simulink model "PSC"  (R2016b)
settings: Solver=VariableStepAuto  StartTime=0.0  StopTime=5  RelTol=1e-3
values from neighbouring files (symbols this model uses):
  A = 1.3    [PV_module_Code.m]
  Isc = 8.61    [PV_module_Code.m]
  Ki = 0.002    [PV_module_Code.m]
  Kv = -0.32    [PV_module_Code.m]
  Ns = 60    [PV_module_Code.m]
  Rp = 415    [PV_module_Code.m]
  Rs = 0.22    [PV_module_Code.m]
  Voc = 37.41    [PV_module_Code.m]
undefined symbols (not defined in the file or in its folder): sigbuilder_block
libraries: powerlib x26, powerlib_meascontrol x1, fuzblock x1
settings Model: Creator=adria  LastModifiedBy=adria
settings DebuggingCC: UnconnectedInputMsg=none  UnconnectedOutputMsg=none  UnconnectedLineMsg=none

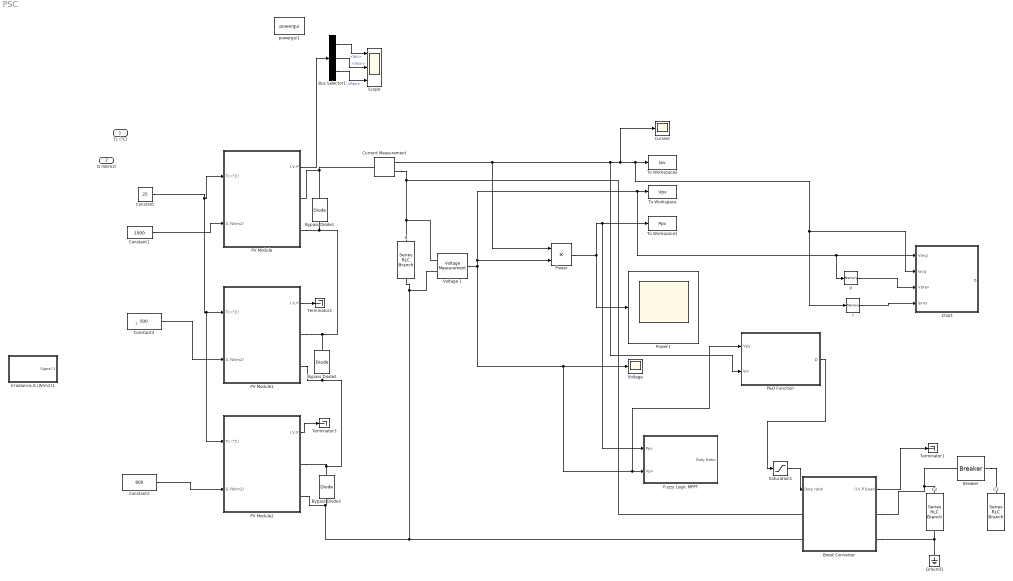
== system PSC ==
  note: 1
  Tc (°C) : Inport
  G (W/m2) : Inport  Port=2
  Boost Converter : Subsystem
  Breaker : powerlib/Elements/Breaker  InitialState=0  SwitchingTimes=[7]  External=off  BreakerResistance=0.00001  SnubberResistance=1e6  SnubberCapacitance=inf  Measurements=None  MoreParameters=on  NoBreakLoop=off
  Bus Selector1 : BusSelector  OutputSignals=Ipv,Vpv,Ppv
  Bypass Diode1 : powerlib/Power Electronics/Diode  Ron=0.00001  Lon=0  Vf=0.8  IC=0  UseSnubber=off  Rs=500  Cs=250e-9  Measurements=off
  Bypass Diode2 : powerlib/Power Electronics/Diode  Ron=0.00001  Lon=0  Vf=0.8  IC=0  UseSnubber=off  Rs=500  Cs=250e-9  Measurements=off
  Bypass Diode3 : powerlib/Power Electronics/Diode  Ron=0.00001  Lon=0  Vf=0.8  IC=0  UseSnubber=off  Rs=500  Cs=250e-9  Measurements=off
  C : powerlib/Elements/Series RLC Branch  LConnTagsString=__new0  RConnTagsString=__new0  BranchType=C  Resistance=3.7  Inductance=1e-3  SetiL0=off  InitialCurrent=0  Capacitance=50e-4  Setx0=off  InitialVoltage=0  Measurements=Branch voltage
  C2 : powerlib/Elements/Series RLC Branch  LConnTagsString=__new0  RConnTagsString=__new0  BranchType=R  Resistance=10  Inductance=1e-3  SetiL0=off  InitialCurrent=0  Capacitance=19e-4  Setx0=off  InitialVoltage=0  Measurements=Branch voltage
  C3 : powerlib/Elements/Series RLC Branch  LConnTagsString=__new0  RConnTagsString=__new0  BranchType=R  Resistance=100  Inductance=1e-3  SetiL0=off  InitialCurrent=0  Capacitance=19e-4  Setx0=off  InitialVoltage=0  Measurements=Branch voltage
  Chart : Stateflow chart  TreatAsAtomicUnit=on
  Constant : Constant  Value=25
  Constant1 : Constant  Value=1000
  Constant2 : Constant  Value=800
  Constant3 : Constant  Value=500
  Current : Scope
  Current Measurement : powerlib/Measurements/Current Measurement  PhasorSimulation=off  OutputType=Complex  PSBequivalent=0
  Fuzzy Logic MPPT : Subsystem
  Ground1 : powerlib/Elements/Ground  LConnTagsString=a
  I : Memory
  Irradiance,G (W/m2)1 : Subsystem  Tag=STV Subsys  LoadFcn=sigbuilder_block('load');  StartFcn=sigbuilder_block('start');  StopFcn=sigbuilder_block('stop');  ClipboardFcn=sigbuilder_block('clipboard');  mask(Sigbuilder block){tuvar=[0:10]}
      mask help: Simulink:masks:SigbuilderBlock_MD
      mask init:
      | if ~strcmp(get_param(bdroot(gcbh),'SimulationStatus'),'stopped') tuvar = sigbuilder_block('maskInit'); end
      settings: CopyFcn=sigbuilder_block('copy');  DeleteFcn=sigbuilder_block('delete');  ModelCloseFcn=sigbuilder_block('modelClose');  PreSaveFcn=sigbuilder_block('preSave');  PauseFcn=sigbuilder_block('pause');  ContinueFcn=sigbuilder_block('continue');  NameChangeFcn=sigbuilder_block('namechange');  OpenFcn=sigbuilder_block('open',[484.8 30.6 470.4 453 ]);  CloseFcn=sigbuilder_block('close');
      mask Display: plot(0, 0, 100, 100,[2, 2, 32, 32, 2], [68, 8, 8, 68, 68],[32, 2], [38, 38], [32, 19, 2],[53, 60, 44], [32, 17, 17, 2],[16, 16, 31, 31]);txt = getActiveGroup(gcbh);text(2, 100, txt,'verticalAlignment', 'top');
  P&O Function : MATLAB Function  TreatAsAtomicUnit=on
  PV Module : Subsystem
  PV Module1 : Subsystem
  PV Module2 : Subsystem
  Power : Product
  Power1 : Scope
  Saturation1 : Saturate  UpperLimit=1  LowerLimit=0.001  ZeroCross=off
  Scope : Scope  NumInputPorts=3
  Terminator1 : Terminator
  Terminator2 : Terminator
  Terminator3 : Terminator
  To Workspace : ToWorkspace  VariableName=Vpv  SampleTime=-1
  To Workspace1 : ToWorkspace  VariableName=Ppv  SampleTime=-1
  To Workspace2 : ToWorkspace  VariableName=Ipv  SampleTime=-1
  V : Memory
  Voltage : Scope
  Voltage 1 : powerlib/Measurements/Voltage Measurement  PhasorSimulation=off  OutputType=Complex  PSBequivalent=0
  powergui1 : powerlib/powergui  Priority=1  SimulationMode=Discrete  SolverType=Tustin/Backward Euler (TBE)  SampleTime=0.00001  frequency=60  SPID=off  DisableSnubberDevices=off  DisableRonSwitches=off  DisableVfSwitches=off  SwTol=0  DisplayEquations=off  Interpol=off  ExternalGateDelay=off  methode=off  Ts=10  FunctionMessages=off  echomessages=off  HookPort=off  EnableUseOfTLC=off  x0status=blocks  frequencyindice=0  Pbase=100e6  ErrMax=1e-4  Iterations=50  UnitsV=kV  UnitsW=MW  buscounter=0  RestoreLinks=warning  ResistiveCurrentMeasurement=off  Frange=[0:2:500]  Ylog=off  Xlog=on  ShowGrid=off  save=off  variable=ZData  structure=0  ZoomFFT=off  StartTime=0.0  cycles=1  DisplayStyle=1  fundamental=60  FreqAxis=off  MaxFrequency=1000  frequencyindicesteady=1  RmsSteady=1  display=off
  wires:
  PV Module/1(I,V,P) -> Bus Selector1/1
  Constant/1 -> PV Module2/1(Tc (°C)), PV Module1/1(Tc (°C)), PV Module/1(Tc (°C))
  Constant1/1 -> PV Module/2(G (W/m2))
  Bus Selector1/2 -> Scope/2  "<Vpv>"
  Bus Selector1/3 -> Scope/3  "<Ppv>"
  Bus Selector1/1 -> Scope/1  "<Ipv>"
  PV Module1/1(I,V,P) -> Terminator2/1
  Current Measurement/1 -> Power/1, P&O Function/2(Ipv), Current/1, Chart/2(Iavg), I/1, To Workspace2/1
  Boost Converter/1((I,V,P)Load) -> Terminator1/1
  Power/1 -> Fuzzy Logic MPPT/1(Ppv), To Workspace1/1, Power1/1
  V/1 -> Chart/3(Vprev)
  I/1 -> Chart/4(Iprev)
  Voltage 1/1 -> Power/2, Chart/1(Vavg), V/1, To Workspace/1, P&O Function/1(Vpv), Fuzzy Logic MPPT/2(Vpv), Voltage/1
  Constant3/1 -> PV Module1/2(G (W/m2))
  PV Module2/1(I,V,P) -> Terminator3/1
  Constant2/1 -> PV Module2/2(G (W/m2))
  Saturation1/1 -> Boost Converter/1("Duty ratio ")
  P&O Function/1(D) -> Saturation1/1
  connections:
  PV Module/RConn2 -- Bypass Diode1/LConn1 -- Bypass Diode2/RConn1 -- PV Module1/RConn1
  PV Module/RConn1 -- Bypass Diode1/RConn1 -- Current Measurement/LConn1
  Voltage 1/LConn1 -- Boost Converter/LConn1 -- Current Measurement/RConn1 -- C/LConn1
  Boost Converter/RConn2 -- C2/RConn1 -- Ground1/LConn1
  Boost Converter/RConn1 -- Breaker/LConn1 -- C2/LConn1
  Breaker/RConn1 -- C3/LConn1
  PV Module2/RConn2 -- Boost Converter/LConn2 -- Voltage 1/LConn2 -- C/RConn1 -- Bypass Diode3/LConn1
  PV Module2/RConn1 -- Bypass Diode2/LConn1 -- PV Module1/RConn2 -- Bypass Diode3/RConn1

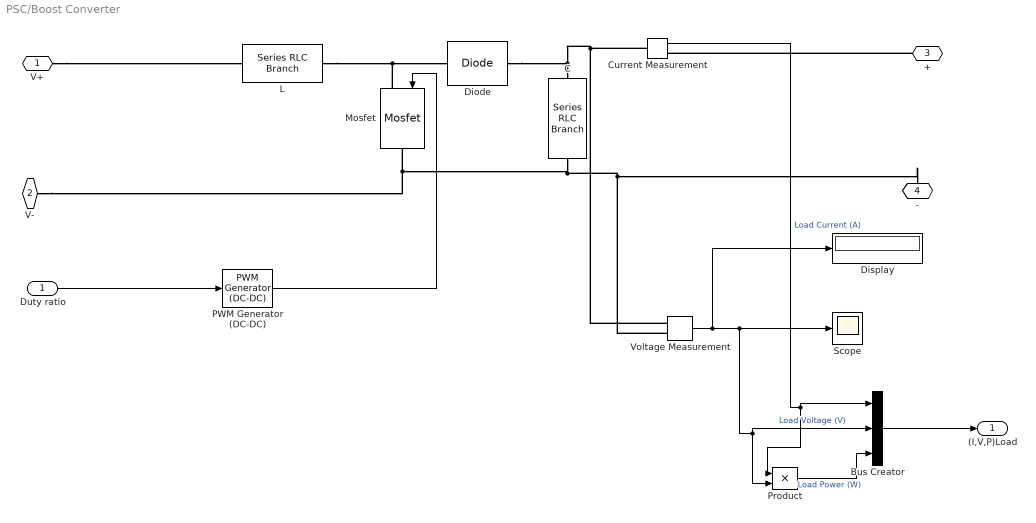
== system PSC/Boost Converter ==
  "Duty ratio " : Inport
  Bus Creator : BusCreator  Inputs='Load Current (A)','Load Voltage (V)','Load Power (W)'
  C : powerlib/Elements/Series RLC Branch  LConnTagsString=__new0  RConnTagsString=__new0  BranchType=C  Resistance=1  Inductance=1e-3  SetiL0=off  InitialCurrent=0  Capacitance=80e-7  Setx0=off  InitialVoltage=0  Measurements=None
  Current Measurement : powerlib/Measurements/Current Measurement  PhasorSimulation=off  OutputType=Complex  PSBequivalent=0
  Diode : powerlib/Power Electronics/Diode  Ron=0.0001  Lon=0  Vf=0.8  IC=0  UseSnubber=off  Rs=500  Cs=250e-9  Measurements=off
  Display : Display
  L : powerlib/Elements/Series RLC Branch  LConnTagsString=__new0  RConnTagsString=__new0  BranchType=L  Resistance=1  Inductance=1e-3  SetiL0=off  InitialCurrent=0  Capacitance=1e-6  Setx0=off  InitialVoltage=0  Measurements=None
  Mosfet : powerlib/Power Electronics/Mosfet  Ron=0.0001  Lon=0  Rd=0.0001  Vfd=0  IC=0  Rs=1e5  Cs=inf  Measurements=off
  PWM Generator (DC-DC) : powerlib_meascontrol/Pulse & Signal Generators/PWM Generator (DC-DC)  Fsw=1000  Ts=0
  Product : Product
  Scope : Scope
  Voltage Measurement : powerlib/Measurements/Voltage Measurement  PhasorSimulation=off  OutputType=Complex  PSBequivalent=0
  V+ : PMIOPort  Port=1  Side=Left
  V- : PMIOPort  Port=2  Side=Left
  + : PMIOPort  Port=3  Side=Right
  - : PMIOPort  Port=4  Side=Right
  (I,V,P)Load : Outport
  wires:
  PWM Generator (DC-DC)/1 -> Mosfet/1
  Voltage Measurement/1 -> Display/1, Product/2, Bus Creator/2, Scope/1  "Load Voltage (V)"
  "Duty ratio "/1 -> PWM Generator (DC-DC)/1
  Current Measurement/1 -> Product/1, Bus Creator/1  "Load Current (A)"
  Product/1 -> Bus Creator/3  "Load Power (W)"
  Bus Creator/1 -> (I,V,P)Load/1
  connections:
  V+/RConn1 -- L/LConn1
  L/RConn1 -- Mosfet/LConn1 -- Diode/LConn1
  +/RConn1 -- Current Measurement/RConn1
  -/RConn1 -- Voltage Measurement/LConn2 -- V-/RConn1 -- Mosfet/RConn1 -- C/RConn1
  Diode/RConn1 -- Current Measurement/LConn1 -- Voltage Measurement/LConn1 -- C/LConn1

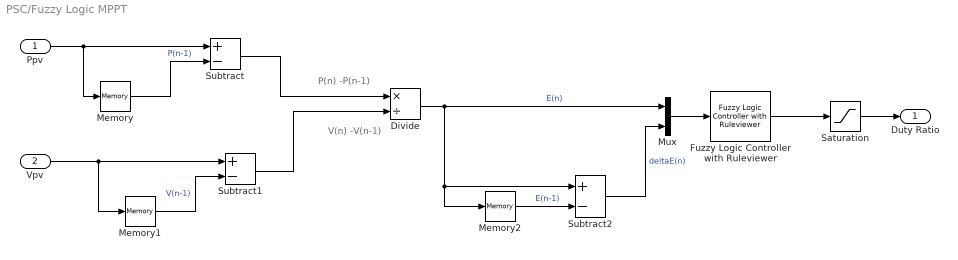
== system PSC/Fuzzy Logic MPPT ==
  note: P(n) -P(n-1)
  note: V(n) -V(n-1)
  Ppv : Inport
  Vpv : Inport  Port=2
  Divide : Product  Inputs=*/
  Fuzzy Logic Controller with Ruleviewer : fuzblock/Fuzzy Logic  Controller  with Ruleviewer  fismatrix=MPPT7  Ts=1
  Memory : Memory
  Memory1 : Memory
  Memory2 : Memory
  Mux : Mux  Inputs=2
  Saturation : Saturate  UpperLimit=1  LowerLimit=0  LinearizeAsGain=off  ZeroCross=off
  Subtract : Sum  Inputs=+-
  Subtract1 : Sum  Inputs=+-
  Subtract2 : Sum  Inputs=+-
  Duty Ratio : Outport
  wires:
  Ppv/1 -> Subtract/1, Memory/1
  Mux/1 -> Fuzzy Logic Controller with Ruleviewer/1
  Divide/1 -> Subtract2/1, Memory2/1, Mux/1  "E(n)"
  Memory2/1 -> Subtract2/2  "E(n-1)"
  Subtract2/1 -> Mux/2  "deltaE(n)"
  Memory/1 -> Subtract/2  "P(n-1)"
  Vpv/1 -> Memory1/1, Subtract1/1
  Memory1/1 -> Subtract1/2  "V(n-1)"
  Saturation/1 -> Duty Ratio/1
  Subtract1/1 -> Divide/2
  Subtract/1 -> Divide/1
  Fuzzy Logic Controller with Ruleviewer/1 -> Saturation/1

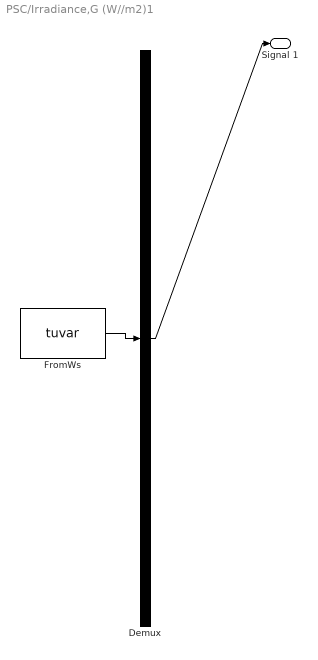
== system PSC/Irradiance,G (W//m2)1 ==
  Demux : Demux  Tag=STV Demux  Outputs=1
  FromWs : FromWorkspace  Tag=STV FromWs  VariableName=tuvar  SampleTime=0
      SigBuilderData=|
      | common.afterFinalStr = 'Extrapolate'
      | common.sampleTime = 0
      | dataSet.timeRange = [0 10]
      | dataSet.name = 'Irradiance Variation Pattern'
      | sbobj.Groups.Name = 'Irradiance Variation Pattern'
      | sbobj.Groups.Signals.Name = 'Signal 1'
      | sbobj.Groups.Signals.XData = [0 0.2 0.2 0.3 0.3 0.8 0.8 0.9 2.4 2.4 3.6 3.6 10]
      | sbobj.Groups.Signals.YData = [1000 1000 300 300 1000 1000 995 995 995 575 1 0 0]
  Signal 1 : Outport  Tag=STV Outport
  wires:
  FromWs/1 -> Demux/1
  Demux/1 -> Signal 1/1

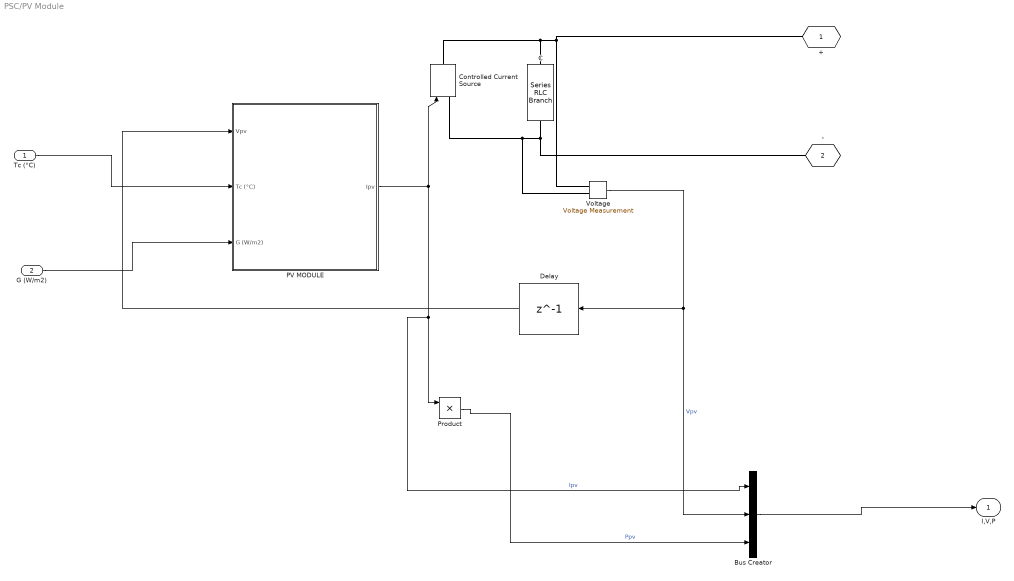
== system PSC/PV Module ==
  Tc (°C) : Inport
  G (W/m2) : Inport  Port=2
  Bus Creator : BusCreator  Inputs='Ipv','Vpv','Ppv'
  C : powerlib/Elements/Series RLC Branch  LConnTagsString=__new0  RConnTagsString=__new0  BranchType=C  Resistance=10  Inductance=1e-3  SetiL0=off  InitialCurrent=0  Capacitance=25e-6  Setx0=off  InitialVoltage=0  Measurements=Branch voltage
  Controlled Current Source : powerlib/Electrical Sources/Controlled Current Source  Initialize=on  Source_Type=AC  Amplitude=0  Phase=0  Frequency=0  Measurements=None
  Delay : Delay  DelayLength=1  InitialCondition=0
  PV MODULE : Subsystem
  Product : Product
  "Voltage " : powerlib/Measurements/Voltage Measurement  PhasorSimulation=off  OutputType=Complex  PSBequivalent=0
  + : PMIOPort  Port=1  Side=Right
  - : PMIOPort  Port=2  Side=Right
  I,V,P : Outport
  wires:
  Product/1 -> Bus Creator/3  "Ppv"
  Tc (°C)/1 -> PV MODULE/2("Tc (°C) ")
  G (W/m2)/1 -> PV MODULE/3(G (W/m2))
  "Voltage "/1 -> Bus Creator/2, Delay/1  "Vpv"
  PV MODULE/1(Ipv) -> Controlled Current Source/1, Bus Creator/1, Product/1  "Ipv"
  Bus Creator/1 -> I,V,P/1
  Delay/1 -> PV MODULE/1(Vpv)
  connections:
  Controlled Current Source/LConn1 -- -/RConn1 -- C/RConn1 -- "Voltage "/LConn2
  Controlled Current Source/RConn1 -- C/LConn1 -- +/RConn1 -- "Voltage "/LConn1

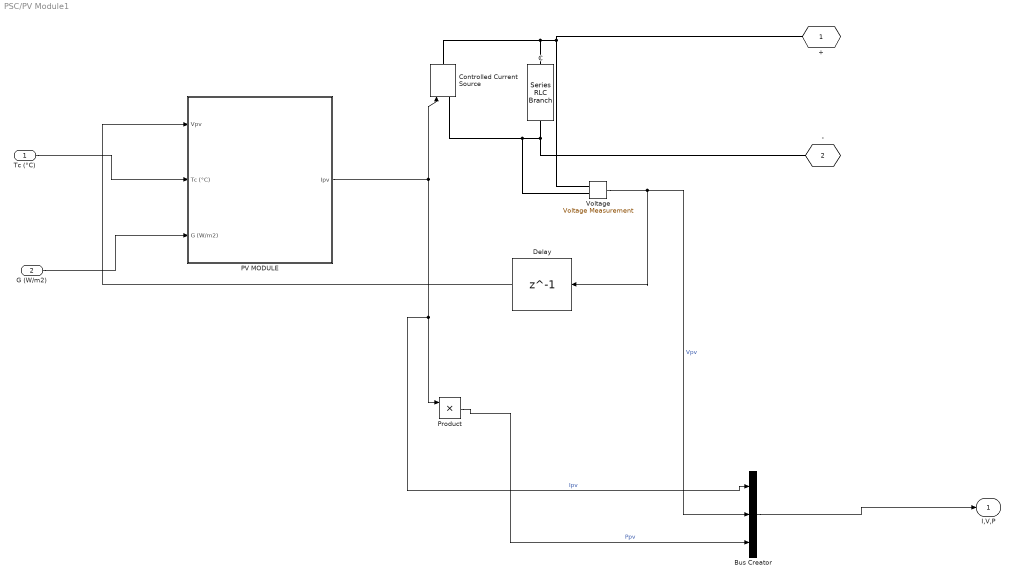
== system PSC/PV Module1 ==
  Tc (°C) : Inport
  G (W/m2) : Inport  Port=2
  Bus Creator : BusCreator  Inputs='Ipv','Vpv','Ppv'
  C : powerlib/Elements/Series RLC Branch  LConnTagsString=__new0  RConnTagsString=__new0  BranchType=C  Resistance=10  Inductance=1e-3  SetiL0=off  InitialCurrent=0  Capacitance=25e-6  Setx0=off  InitialVoltage=0  Measurements=Branch voltage
  Controlled Current Source : powerlib/Electrical Sources/Controlled Current Source  Initialize=on  Source_Type=AC  Amplitude=0  Phase=0  Frequency=0  Measurements=None
  Delay : Delay  DelayLength=1  InitialCondition=0
  PV MODULE : Subsystem
  Product : Product
  "Voltage " : powerlib/Measurements/Voltage Measurement  PhasorSimulation=off  OutputType=Complex  PSBequivalent=0
  + : PMIOPort  Port=1  Side=Right
  - : PMIOPort  Port=2  Side=Right
  I,V,P : Outport
  wires:
  Product/1 -> Bus Creator/3  "Ppv"
  Tc (°C)/1 -> PV MODULE/2("Tc (°C) ")
  G (W/m2)/1 -> PV MODULE/3(G (W/m2))
  "Voltage "/1 -> Delay/1, Bus Creator/2  "Vpv"
  PV MODULE/1(Ipv) -> Bus Creator/1, Product/1, Controlled Current Source/1  "Ipv"
  Bus Creator/1 -> I,V,P/1
  Delay/1 -> PV MODULE/1(Vpv)
  connections:
  Controlled Current Source/LConn1 -- -/RConn1 -- C/RConn1 -- "Voltage "/LConn2
  Controlled Current Source/RConn1 -- C/LConn1 -- +/RConn1 -- "Voltage "/LConn1

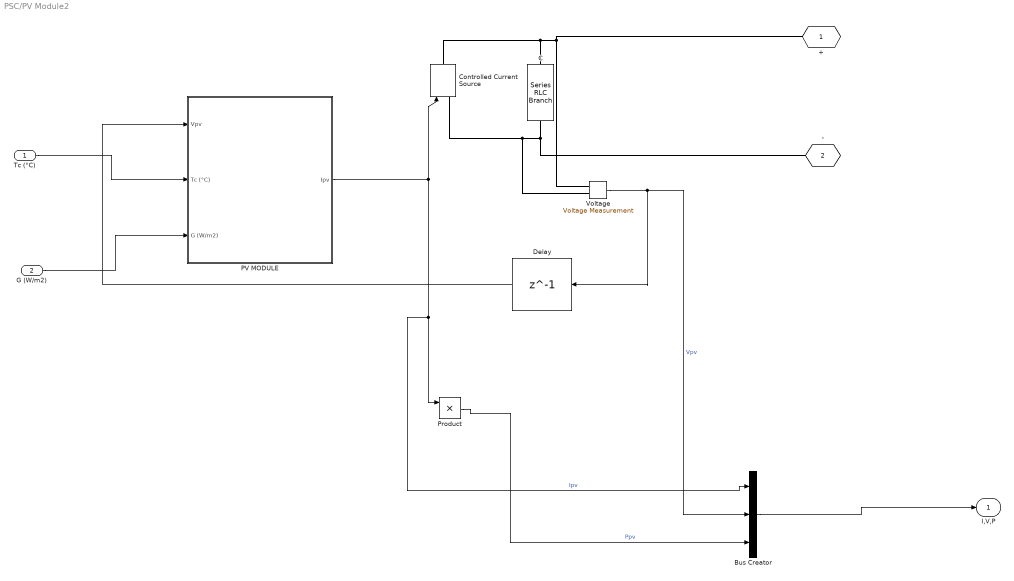
== system PSC/PV Module2 ==
  Tc (°C) : Inport
  G (W/m2) : Inport  Port=2
  Bus Creator : BusCreator  Inputs='Ipv','Vpv','Ppv'
  C : powerlib/Elements/Series RLC Branch  LConnTagsString=__new0  RConnTagsString=__new0  BranchType=C  Resistance=10  Inductance=1e-3  SetiL0=off  InitialCurrent=0  Capacitance=25e-6  Setx0=off  InitialVoltage=0  Measurements=Branch voltage
  Controlled Current Source : powerlib/Electrical Sources/Controlled Current Source  Initialize=on  Source_Type=AC  Amplitude=0  Phase=0  Frequency=0  Measurements=None
  Delay : Delay  DelayLength=1  InitialCondition=0
  PV MODULE : Subsystem
  Product : Product
  "Voltage " : powerlib/Measurements/Voltage Measurement  PhasorSimulation=off  OutputType=Complex  PSBequivalent=0
  + : PMIOPort  Port=1  Side=Right
  - : PMIOPort  Port=2  Side=Right
  I,V,P : Outport
  wires:
  Product/1 -> Bus Creator/3  "Ppv"
  Tc (°C)/1 -> PV MODULE/2("Tc (°C) ")
  G (W/m2)/1 -> PV MODULE/3(G (W/m2))
  "Voltage "/1 -> Delay/1, Bus Creator/2  "Vpv"
  PV MODULE/1(Ipv) -> Bus Creator/1, Product/1, Controlled Current Source/1  "Ipv"
  Bus Creator/1 -> I,V,P/1
  Delay/1 -> PV MODULE/1(Vpv)
  connections:
  Controlled Current Source/LConn1 -- -/RConn1 -- C/RConn1 -- "Voltage "/LConn2
  Controlled Current Source/RConn1 -- C/LConn1 -- +/RConn1 -- "Voltage "/LConn1

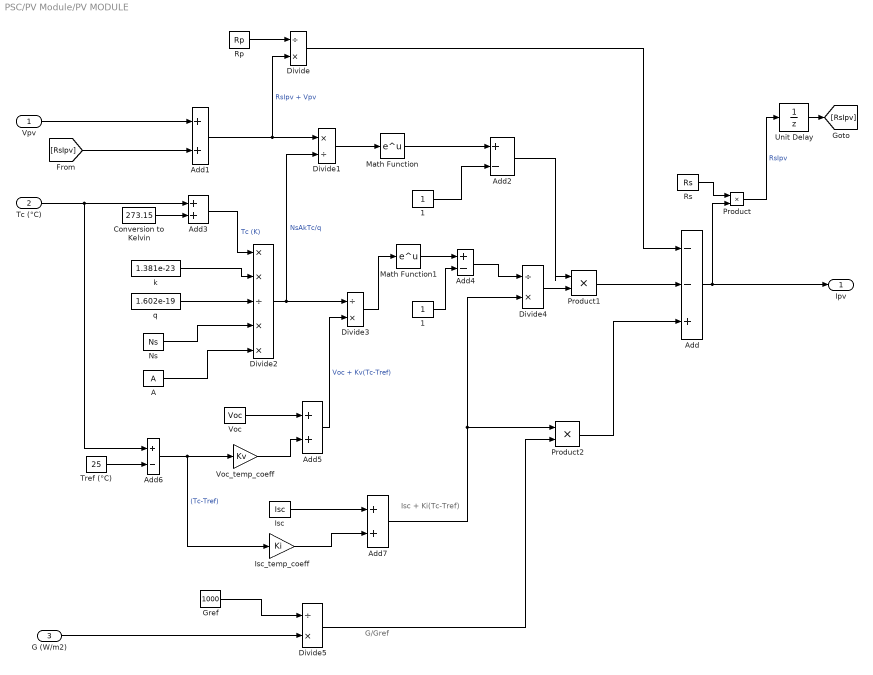
== system PSC/PV Module/PV MODULE ==
  note: G/Gref
  note: Isc + Ki(Tc-Tref)
  Vpv : Inport
  "Tc (°C) " : Inport  Port=2
  G (W/m2) : Inport  Port=3
  " 1" : Constant
  " Gref " : Constant  Value=1000
  " Tref (°C)" : Constant  Value=25
  " Voc" : Constant  Value=Voc
  1 : Constant
  A : Constant  Value=A
  Add : Sum  Inputs=--+
  Add{1,3,5,7} (4 alike) : Sum
  Add2 : Sum  Inputs=+-
  Add4 : Sum  Inputs=+-
  Add6 : Sum  Inputs=+-
  Conversion to Kelvin : Constant  Value=273.15
  Divide{,3..5} (4 alike) : Product  Inputs=/*
  Divide1 : Product  Inputs=*/
  Divide2 : Product  Inputs=**/**
  Isc : Constant  Value=Isc
  "Isc_temp_coeff " : Gain  Gain=Ki
  Math Function : Math  SaturateOnIntegerOverflow=on
  Math Function1 : Math  SaturateOnIntegerOverflow=on
  Ns : Constant  Value=Ns
  Product : Product
  Product1 : Product
  Product2 : Product
  Rp : Constant  Value=Rp
  Rs : Constant  Value=Rs
  Unit Delay : UnitDelay  SampleTime=-1
  Voc_temp_coeff : Gain  Gain=Kv
  k : Constant  Value=1.381e-23
  "q " : Constant  Value=1.602e-19
  Ipv : Outport
  wires:
  A/1 -> Divide2/5
  Vpv/1 -> Add1/1
  Rp/1 -> Divide/1
  Add/1 -> Ipv/1, Product/2
  Product/1 -> Unit Delay/1  "RsIpv"
  Divide/1 -> Add/1
  Add1/1 -> Divide1/1, Divide/2  "RsIpv + Vpv"
  Rs/1 -> Product/1
  Product2/1 -> Add/3
  Divide2/1 -> Divide3/1, Divide1/2  "NsAkTc/q"
  k/1 -> Divide2/2
  Math Function1/1 -> Add4/1
  " Voc"/1 -> Add5/1
  Divide4/1 -> Product1/2
  Add2/1 -> Product1/1
  Math Function/1 -> Add2/1
  Divide3/1 -> Math Function1/1
  "q "/1 -> Divide2/3
  Add6/1 -> "Isc_temp_coeff "/1, Voc_temp_coeff/1  "(Tc-Tref)"
  " 1"/1 -> Add4/2
  Isc/1 -> Add7/1
  Add7/1 -> Product2/1, Divide4/2
  "Tc (°C) "/1 -> Add6/1, Add3/1
  Add4/1 -> Divide4/1
  Product1/1 -> Add/2
  Divide5/1 -> Product2/2
  Conversion to Kelvin/1 -> Add3/2
  Add5/1 -> Divide3/2  "Voc + Kv(Tc-Tref)"
  "Isc_temp_coeff "/1 -> Add7/2
  Divide1/1 -> Math Function/1
  " Gref "/1 -> Divide5/1
  " Tref (°C)"/1 -> Add6/2
  G (W/m2)/1 -> Divide5/2
  Voc_temp_coeff/1 -> Add5/2
  Add3/1 -> Divide2/1  "Tc (K)"
  Ns/1 -> Divide2/4
  1/1 -> Add2/2
  [RsIpv] -> Add1/2
  Unit Delay/1 -> [RsIpv]

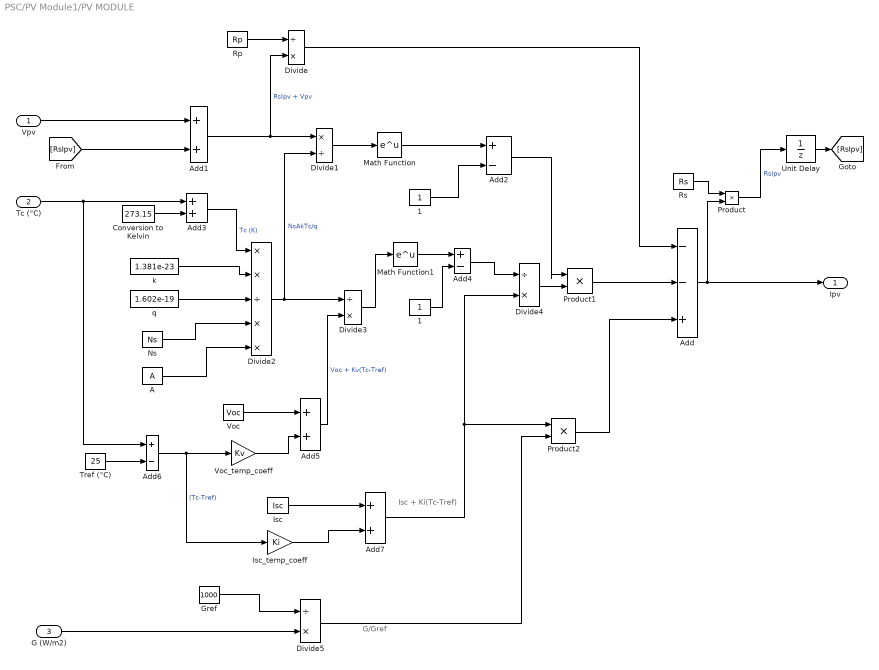
== system PSC/PV Module1/PV MODULE ==
  note: G/Gref
  note: Isc + Ki(Tc-Tref)
  Vpv : Inport
  "Tc (°C) " : Inport  Port=2
  G (W/m2) : Inport  Port=3
  " 1" : Constant
  " Gref " : Constant  Value=1000
  " Tref (°C)" : Constant  Value=25
  " Voc" : Constant  Value=Voc
  1 : Constant
  A : Constant  Value=A
  Add : Sum  Inputs=--+
  Add{1,3,5,7} (4 alike) : Sum
  Add2 : Sum  Inputs=+-
  Add4 : Sum  Inputs=+-
  Add6 : Sum  Inputs=+-
  Conversion to Kelvin : Constant  Value=273.15
  Divide{,3..5} (4 alike) : Product  Inputs=/*
  Divide1 : Product  Inputs=*/
  Divide2 : Product  Inputs=**/**
  Isc : Constant  Value=Isc
  "Isc_temp_coeff " : Gain  Gain=Ki
  Math Function : Math  SaturateOnIntegerOverflow=on
  Math Function1 : Math  SaturateOnIntegerOverflow=on
  Ns : Constant  Value=Ns
  Product : Product
  Product1 : Product
  Product2 : Product
  Rp : Constant  Value=Rp
  Rs : Constant  Value=Rs
  Unit Delay : UnitDelay  SampleTime=-1
  Voc_temp_coeff : Gain  Gain=Kv
  k : Constant  Value=1.381e-23
  "q " : Constant  Value=1.602e-19
  Ipv : Outport
  wires:
  A/1 -> Divide2/5
  Vpv/1 -> Add1/1
  Rp/1 -> Divide/1
  Add/1 -> Ipv/1, Product/2
  Product/1 -> Unit Delay/1  "RsIpv"
  Divide/1 -> Add/1
  Add1/1 -> Divide1/1, Divide/2  "RsIpv + Vpv"
  Rs/1 -> Product/1
  Product2/1 -> Add/3
  Divide2/1 -> Divide3/1, Divide1/2  "NsAkTc/q"
  k/1 -> Divide2/2
  Math Function1/1 -> Add4/1
  " Voc"/1 -> Add5/1
  Divide4/1 -> Product1/2
  Add2/1 -> Product1/1
  Math Function/1 -> Add2/1
  Divide3/1 -> Math Function1/1
  "q "/1 -> Divide2/3
  Add6/1 -> "Isc_temp_coeff "/1, Voc_temp_coeff/1  "(Tc-Tref)"
  " 1"/1 -> Add4/2
  Isc/1 -> Add7/1
  Add7/1 -> Product2/1, Divide4/2
  "Tc (°C) "/1 -> Add6/1, Add3/1
  Add4/1 -> Divide4/1
  Product1/1 -> Add/2
  Divide5/1 -> Product2/2
  Conversion to Kelvin/1 -> Add3/2
  Add5/1 -> Divide3/2  "Voc + Kv(Tc-Tref)"
  "Isc_temp_coeff "/1 -> Add7/2
  Divide1/1 -> Math Function/1
  " Gref "/1 -> Divide5/1
  " Tref (°C)"/1 -> Add6/2
  G (W/m2)/1 -> Divide5/2
  Voc_temp_coeff/1 -> Add5/2
  Add3/1 -> Divide2/1  "Tc (K)"
  Ns/1 -> Divide2/4
  1/1 -> Add2/2
  [RsIpv] -> Add1/2
  Unit Delay/1 -> [RsIpv]

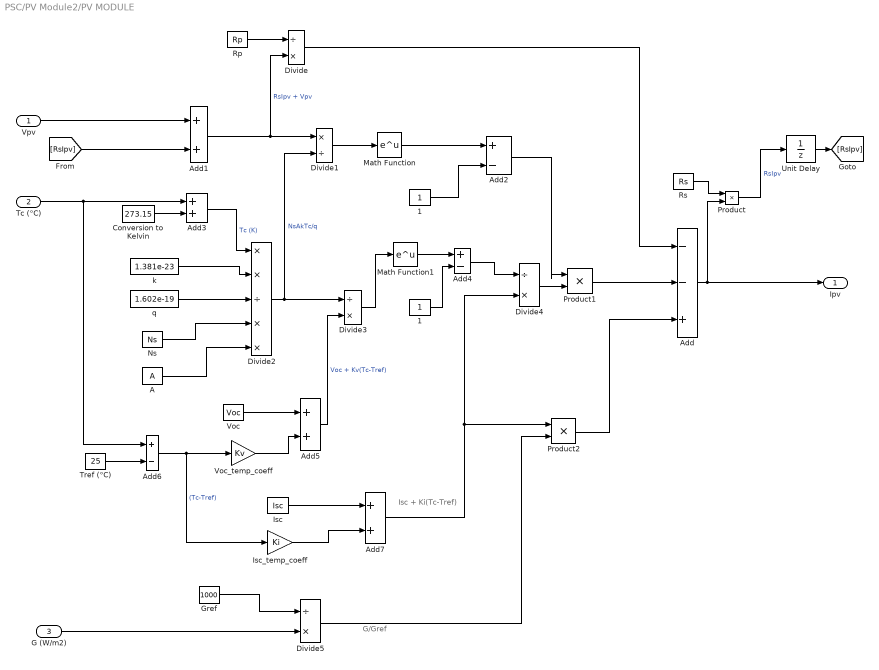
== system PSC/PV Module2/PV MODULE ==
  note: G/Gref
  note: Isc + Ki(Tc-Tref)
  Vpv : Inport
  "Tc (°C) " : Inport  Port=2
  G (W/m2) : Inport  Port=3
  " 1" : Constant
  " Gref " : Constant  Value=1000
  " Tref (°C)" : Constant  Value=25
  " Voc" : Constant  Value=Voc
  1 : Constant
  A : Constant  Value=A
  Add : Sum  Inputs=--+
  Add{1,3,5,7} (4 alike) : Sum
  Add2 : Sum  Inputs=+-
  Add4 : Sum  Inputs=+-
  Add6 : Sum  Inputs=+-
  Conversion to Kelvin : Constant  Value=273.15
  Divide{,3..5} (4 alike) : Product  Inputs=/*
  Divide1 : Product  Inputs=*/
  Divide2 : Product  Inputs=**/**
  Isc : Constant  Value=Isc
  "Isc_temp_coeff " : Gain  Gain=Ki
  Math Function : Math  SaturateOnIntegerOverflow=on
  Math Function1 : Math  SaturateOnIntegerOverflow=on
  Ns : Constant  Value=Ns
  Product : Product
  Product1 : Product
  Product2 : Product
  Rp : Constant  Value=Rp
  Rs : Constant  Value=Rs
  Unit Delay : UnitDelay  SampleTime=-1
  Voc_temp_coeff : Gain  Gain=Kv
  k : Constant  Value=1.381e-23
  "q " : Constant  Value=1.602e-19
  Ipv : Outport
  wires:
  A/1 -> Divide2/5
  Vpv/1 -> Add1/1
  Rp/1 -> Divide/1
  Add/1 -> Ipv/1, Product/2
  Product/1 -> Unit Delay/1  "RsIpv"
  Divide/1 -> Add/1
  Add1/1 -> Divide1/1, Divide/2  "RsIpv + Vpv"
  Rs/1 -> Product/1
  Product2/1 -> Add/3
  Divide2/1 -> Divide3/1, Divide1/2  "NsAkTc/q"
  k/1 -> Divide2/2
  Math Function1/1 -> Add4/1
  " Voc"/1 -> Add5/1
  Divide4/1 -> Product1/2
  Add2/1 -> Product1/1
  Math Function/1 -> Add2/1
  Divide3/1 -> Math Function1/1
  "q "/1 -> Divide2/3
  Add6/1 -> "Isc_temp_coeff "/1, Voc_temp_coeff/1  "(Tc-Tref)"
  " 1"/1 -> Add4/2
  Isc/1 -> Add7/1
  Add7/1 -> Product2/1, Divide4/2
  "Tc (°C) "/1 -> Add6/1, Add3/1
  Add4/1 -> Divide4/1
  Product1/1 -> Add/2
  Divide5/1 -> Product2/2
  Conversion to Kelvin/1 -> Add3/2
  Add5/1 -> Divide3/2  "Voc + Kv(Tc-Tref)"
  "Isc_temp_coeff "/1 -> Add7/2
  Divide1/1 -> Math Function/1
  " Gref "/1 -> Divide5/1
  " Tref (°C)"/1 -> Add6/2
  G (W/m2)/1 -> Divide5/2
  Voc_temp_coeff/1 -> Add5/2
  Add3/1 -> Divide2/1  "Tc (K)"
  Ns/1 -> Divide2/4
  1/1 -> Add2/2
  [RsIpv] -> Add1/2
  Unit Delay/1 -> [RsIpv]

== matlab function PSC/P&O Function ==
  data: Vpv input; D output; Ipv input
function D = PO_Algorithm(Vpv,Ipv)
%P&O algoritm implmentation designed to operate 
%with Boost converter
%************************************
%Created by Joseph Adriano Nemours

%Define Inernal Values for the power nad voltage 
%a persistent variables
persistent Dprev Pprev Vprev

%Initialise the internal vlaues for the voltage 
%and power on the first pass (ot iteration)
if isempty (Dprev)
    Dprev = 0.8;
    Vprev = 0;
    Pprev = 0;
end

%Initialise algoritm parameters
deltaD = 0.001;

%Calculate measured array power
Ppv = Ipv * Vpv;

%Increase or decrease duty cycle 
%based on conditions
if (Ppv-Pprev)~= 0
    if (Ppv-Pprev) > 0
        if (Vpv-Vprev) > 0
            D = Dprev - deltaD;
        else 
            D = Dprev + deltaD;
        end
    else
        if (Vpv-Vprev) > 0
                D = Dprev + deltaD;
        else
            D = Dprev - deltaD;
        end
    end
else
    D = Dprev;
end
if D >= 0.8 || D<= 0
 D=Dprev;
end

%Update internal value of Duty ratio
Dprev = D;
Pprev = Ppv;
Vprev = Vpv;

== stateflow chart PSC/Chart ==
  state DEFINE
    entry: D=0.8;
  state SAMPLEandCALCULATE
    entry:
    deltaV = Vavg-Vprev;
    deltaI = Iavg - Iprev;
    d=D;
  state INCREMENT_D
    entry:
    d = d + 0.001;
  state DECREMENT_D
    entry:
    d = d - 0.001;
  state RETURN
    entry:
    D = d;
  (default) -> DEFINE
  RETURN -> SAMPLEandCALCULATE
  DEFINE -> SAMPLEandCALCULATE
  SAMPLEandCALCULATE -> (junction 14) [order 1] : [deltaV==0]
  SAMPLEandCALCULATE -> (junction 13) [order 2] : [deltaV~=0]
  (junction 13) -> DECREMENT_D [order 1] : [deltaI/deltaV>-Iavg/Vavg]
  (junction 13) -> RETURN [order 3] : [deltaI/deltaV==-Iavg/Vavg]
  (junction 13) -> INCREMENT_D [order 2] : [deltaI/deltaV<-Iavg/Vavg]
  (junction 14) -> INCREMENT_D [order 1] : [deltaI<0]
  (junction 14) -> RETURN [order 3] : [deltaI==0]
  (junction 14) -> DECREMENT_D [order 2] : [deltaI>0]
  DECREMENT_D -> RETURN
  INCREMENT_D -> RETURN
  data: deltaI local double; k local; deltaV local; Vavg input; Iavg input; Vprev input; Iprev input; d local double; D output
